simulink model "BicyclePeterCorkePathFollow"  (R2021a)
settings: Solver=VariableStepAuto  StartTime=0.0  StopTime=1000  RelTol=1e-3
undefined symbols (not defined in the file): accelLim, initCoord, lookaheadDist, path, speedLim, steerLim, wheelBase
libraries: robotalgslib x1, simulink x1
settings Model: Creator=User  LastModifiedBy=User

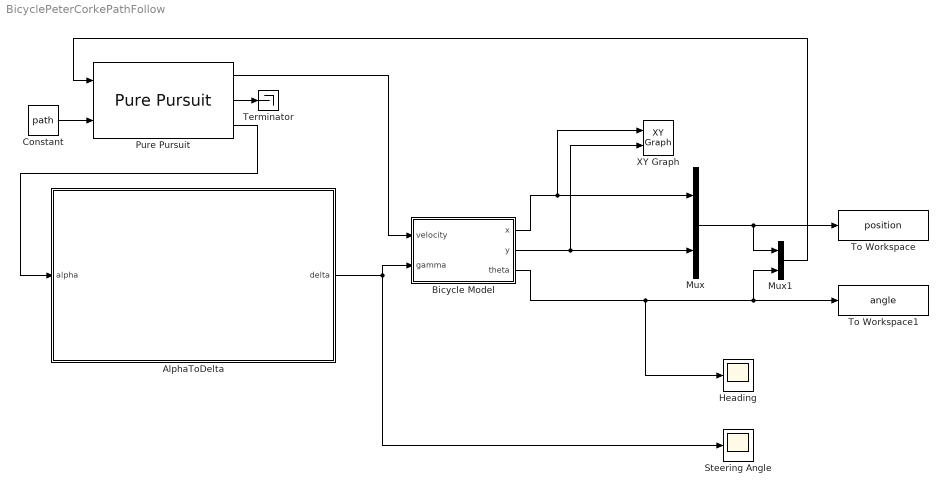
== system BicyclePeterCorkePathFollow ==
  AlphaToDelta : Subsystem
  Bicycle Model : Subsystem
  Constant : Constant  Value=path
  Heading : Scope
  Mux : Mux  Inputs=2
  Mux1 : Mux  Inputs=2
  Pure Pursuit : robotalgslib/Pure Pursuit  DesiredLinearVelocity=0.1  MaxAngularVelocity=1  LookaheadDistance=lookaheadDist  TargetDirPort=on  SimulateUsing=Code generation
  Steering Angle : Scope
  Terminator : Terminator
  To Workspace : ToWorkspace  VariableName=position  SaveFormat=Timeseries  SampleTime=-1
  To Workspace1 : ToWorkspace  VariableName=angle  SaveFormat=Timeseries  SampleTime=-1
  XY Graph : simulink/Sinks/XY Graph  xmin=-10  xmax=10  ymin=-10  ymax=10  st=-1
  wires:
  Bicycle Model/2(y) -> Mux/2, XY Graph/2
  Bicycle Model/1(x) -> Mux/1, XY Graph/1
  Mux/1 -> Mux1/1, To Workspace/1
  Bicycle Model/3(theta) -> Mux1/2, To Workspace1/1, Heading/1
  AlphaToDelta/1(delta) -> Steering Angle/1, Bicycle Model/2(gamma)
  Pure Pursuit/1 -> Bicycle Model/1(velocity)
  Mux1/1 -> Pure Pursuit/1
  Constant/1 -> Pure Pursuit/2
  Pure Pursuit/2 -> Terminator/1
  Pure Pursuit/3 -> AlphaToDelta/1(alpha)

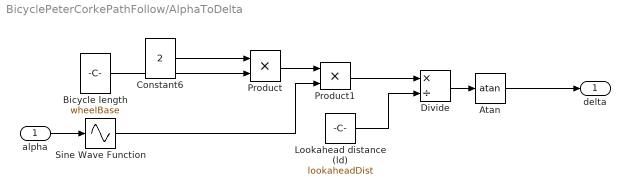
== system BicyclePeterCorkePathFollow/AlphaToDelta ==
  alpha : Inport
  Atan : Trigonometry  Operator=atan
  Bicycle length : Constant  Value=wheelBase  VectorParams1D=off
  Constant6 : Constant  Value=2  VectorParams1D=off
  Divide : Product  Inputs=*/
  Lookahead distance (ld) : Constant  Value=lookaheadDist  VectorParams1D=off
  Product : Product
  Product1 : Product
  Sine Wave Function : Sin  TimeSource=Use external signal  SampleTime=0
  delta : Outport
  wires:
  Lookahead distance (ld)/1 -> Divide/2
  Atan/1 -> delta/1
  Sine Wave Function/1 -> Product1/2
  Product/1 -> Product1/1
  alpha/1 -> Sine Wave Function/1
  Divide/1 -> Atan/1
  Bicycle length/1 -> Product/2
  Constant6/1 -> Product/1
  Product1/1 -> Divide/1

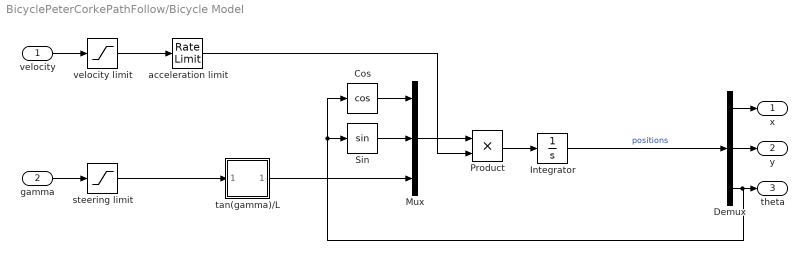
== system BicyclePeterCorkePathFollow/Bicycle Model ==
  velocity : Inport
  gamma : Inport  Port=2
  Cos : Trigonometry  Operator=cos
  Demux : Demux  Outputs=3
  Integrator : Integrator  InitialCondition=initCoord
  Mux : Mux  Inputs=3
  Product : Product
  Sin : Trigonometry
  acceleration limit : RateLimiter  RisingSlewLimit=accelLim  FallingSlewLimit=-accelLim  SampleTimeMode=inherited
  steering limit : Saturate  UpperLimit=steerLim  LowerLimit=-steerLim
  tan(gamma)/L : Subsystem
  velocity limit : Saturate  UpperLimit=speedLim  LowerLimit=-speedLim
  x : Outport
  y : Outport  Port=2
  theta : Outport  Port=3
  wires:
  velocity/1 -> velocity limit/1
  velocity limit/1 -> acceleration limit/1
  gamma/1 -> steering limit/1
  steering limit/1 -> tan(gamma)/L/1(In1)
  tan(gamma)/L/1(Out1) -> Mux/3
  Mux/1 -> Product/1
  acceleration limit/1 -> Product/2
  Product/1 -> Integrator/1
  Integrator/1 -> Demux/1  "positions"
  Demux/3 -> Cos/1, Sin/1, theta/1
  Demux/1 -> x/1
  Demux/2 -> y/1
  Cos/1 -> Mux/1
  Sin/1 -> Mux/2

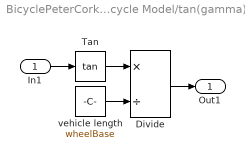
== system BicyclePeterCorkePathFollow/Bicycle Model/tan(gamma)//L ==
  In1 : Inport
  Divide : Product  Inputs=*/
  Tan : Trigonometry  Operator=tan
  vehicle length : Constant  Value=wheelBase
  Out1 : Outport
  wires:
  Tan/1 -> Divide/1
  vehicle length/1 -> Divide/2
  In1/1 -> Tan/1
  Divide/1 -> Out1/1
